simulink model "subsistema_mecanico"  (R2023b)
settings: Solver=VariableStepAuto  StartTime=0.0  StopTime=10.0  RelTol=1e-3
values from neighbouring files (symbols this model uses):
  beq_nom = bm + bl_nom/r^2    (= 2.19444444444e-05)    [parametros_planta.m]    (also in params_subsistema_mecanico.m; sistema_completo_en_codigo.m)
  Jeq_nom = Jm + Jl_nom/r^2    (= 1.97847222222e-05)    [params_subsistema_mecanico.m]    (also in sistema_completo_en_codigo.m)
  kg_eq_nom = g*kl_nom/r    (= 0.0204305208333)    [params_subsistema_mecanico.m]    (also in sistema_completo_en_codigo.m)
  r = 120.0    (= 120)    [controlador_foc_simulink.m]    (also in parametros_planta.m; params_subsistema_mecanico.m; sistema_completo_en_codigo.m)
settings Model: Creator=Gabriel  LastModifiedBy=Pc

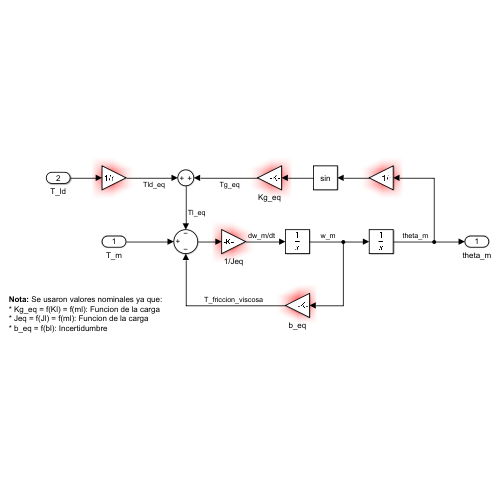
[thumbnail: Simulink's stored preview of the top-level diagram]
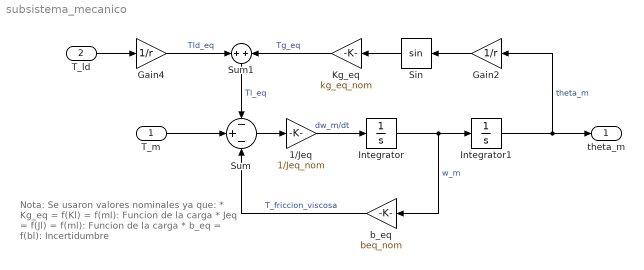
== system subsistema_mecanico ==
  note: Nota: Se usaron valores nominales ya que:
      | * Kg_eq = f(Kl) = f(ml): Funcion de la carga
      | * Jeq = f(Jl) = f(ml): Funcion de la carga
      | * b_eq = f(bl): Incertidumbre
  T_m : Inport
  T_ld : Inport  Port=2
  1/Jeq : Gain  Gain=1/Jeq_nom
  Gain2 : Gain  Gain=1/r
  Gain4 : Gain  Gain=1/r
  Integrator : Integrator
  Integrator1 : Integrator
  Kg_eq : Gain  Gain=kg_eq_nom
  Sin : Trigonometry
  Sum : Sum  Inputs=-+-
  Sum1 : Sum  Inputs=+|+
  b_eq : Gain  Gain=beq_nom
  theta_m : Outport
  wires:
  Integrator1/1 -> Gain2/1, theta_m/1  "theta_m"
  Sum/1 -> 1/Jeq/1
  1/Jeq/1 -> Integrator/1  "dw_m/dt"
  Integrator/1 -> b_eq/1, Integrator1/1  "w_m"
  Gain2/1 -> Sin/1
  Sin/1 -> Kg_eq/1
  T_ld/1 -> Gain4/1
  T_m/1 -> Sum/2
  b_eq/1 -> Sum/3  "T_friccion_viscosa"
  Kg_eq/1 -> Sum1/2  "Tg_eq"
  Gain4/1 -> Sum1/1  "Tld_eq"
  Sum1/1 -> Sum/1  "Tl_eq"
